simulink model "PolarCinematica"  (R2022a)
settings: Solver=VariableStepAuto  StartTime=0.0  StopTime=Tfinal  RelTol=1e-3
values from neighbouring files (symbols this model uses):
  Tem = 0.001    [circular.m]
undefined symbols (not defined in the file or in its folder): Diferencia, mgd_Polar, mgi_Polar
settings Model: Creator=Shadow  LastModifiedBy=Shadow
settings DebuggingCC: UnconnectedInputMsg=warning  UnconnectedOutputMsg=warning  UnconnectedLineMsg=warning
settings RTWCC: DLArmComputeVersion=19.05

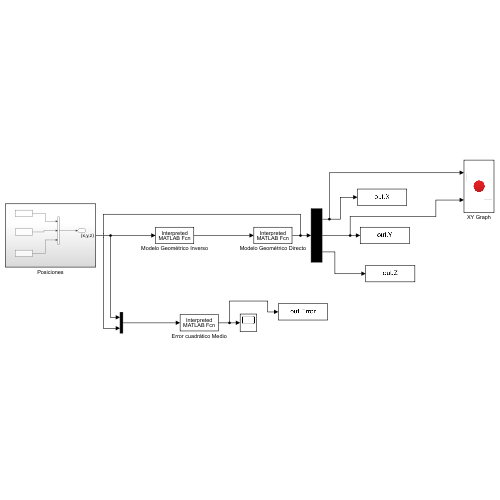
[thumbnail: Simulink's stored preview of the top-level diagram]
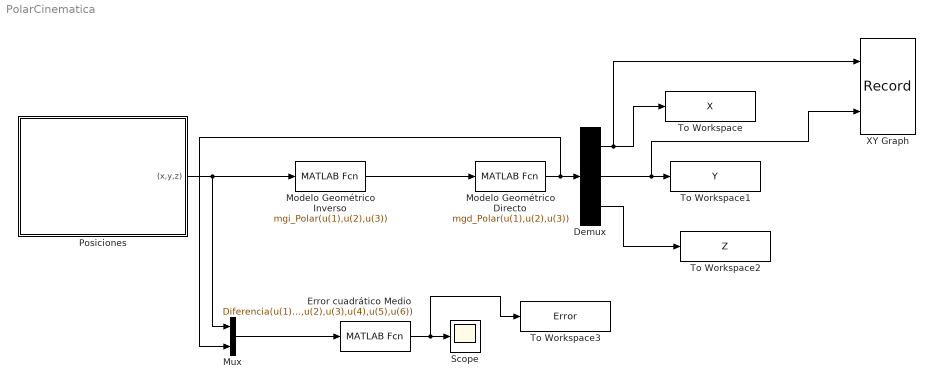
== system PolarCinematica ==
  Demux : Demux  Outputs=3
  Error cuadrático Medio : MATLABFcn  MATLABFcn=Diferencia(u(1),u(2),u(3),u(4),u(5),u(6))  OutputDimensions=1
  Modelo Geométrico Directo : MATLABFcn  MATLABFcn=mgd_Polar(u(1),u(2),u(3))  OutputDimensions=3
  Modelo Geométrico Inverso : MATLABFcn  MATLABFcn=mgi_Polar(u(1),u(2),u(3))  OutputDimensions=3
  Mux : Mux  Inputs=2
  Posiciones : Subsystem
  Scope : Scope
  To Workspace : ToWorkspace  VariableName=X
  To Workspace1 : ToWorkspace  VariableName=Y
  To Workspace2 : ToWorkspace  VariableName=Z
  To Workspace3 : ToWorkspace  VariableName=Error
  XY Graph : Record  FileSettingsInternal="{\"entries\":[{\"content\":{\"excelSettings\":{\"content\":{},\"type\":\"Streamout.ExcelSettings\"}},\"type\":\"Streamout.FileSettingStorage\",\"uuid\":\"bcd1633b-806b-4dc5-b82f-7056fa3f72c6\"}],\"packageUris\":[\"http://schema.mathworks.com/mf0/streamout_blocks/R2020a\"],\"version\":\"1.0\"}"  Layout=[1 1]  SignalsInternal="{\"entries\":[{\"content\":{\"signals\":[{\"content\":{\"blockPath\":[\"PolarCinematica/XY Graph\"],\"channel\":[],\"dimensions\":[1],\"domain\":\"PolarCinematica/XY Graph\",\"lineColor\":\"#a2142f\",\"plots\":[1],\"port\":1,\"sid\":[\"\"],\"signalID\":28,\"signalName\":\"Demux:1\"},\"type\":\"RecordBlkView.Signal\",\"uuid\":\"7db50e9b-d9aa-4afa-8b6e-b476f31eaf6f\"},{\"content\":{\"blockPath\":[\"PolarCinematica/XY Graph\"],\"channel\":[],\"dimensions\":[1],\"domain\":\"PolarCinematica/XY Graph\",\"lineColor\":\"#139fff\",\"plots\":[1],\"port\":2,\"sid\":[\"\"],\"signalID\":32,\"signalName\":\"Demux:2\"},\"type\":\"RecordBlkView.Signal\",\"uuid\":\"48e31d0b-9318-448c-a423-086d85bbcbc5\"}]},\"type\":\"RecordBlkView.InputSignals\",\"uuid\":\"946ceb7c-b64a-43a8-9baa-8683f0c128d2\"}],\"packageUris\":[\"http://schema.mathworks.com/mf0/streamout_blocks/R2020a\"],\"version\":\"1.0\"}"  VisualizationBindings="{\"xyplotplugin\":{\"info\":[{\"series\":[{\"bindingParametersList\":[{\"parameter\":\"X-Axis\",\"signalID\":28,\"signalName\":\"Demux:1\"},{\"parameter\":\"Y-Axis\",\"signalID\":32,\"signalName\":\"Demux:2\"}],\"seriesID\":43994}],\"subplotID\":1}]}}"  CompatibilityTag=XY
  wires:
  Demux/2 -> XY Graph/2, To Workspace1/1
  Demux/3 -> To Workspace2/1
  Modelo Geométrico Inverso/1 -> Modelo Geométrico Directo/1
  Posiciones/1((x,y,z)) -> Mux/1, Modelo Geométrico Inverso/1
  Demux/1 -> To Workspace/1, XY Graph/1
  Mux/1 -> Error cuadrático Medio/1
  Modelo Geométrico Directo/1 -> Mux/2, Demux/1
  Error cuadrático Medio/1 -> To Workspace3/1, Scope/1

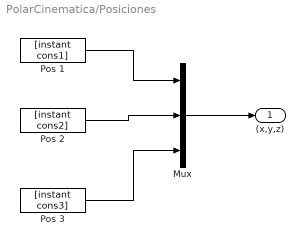
== system PolarCinematica/Posiciones ==
  Mux : Mux  Inputs=3
  Pos 1 : FromWorkspace  VariableName=[instant cons1]  SampleTime=Tem
  Pos 2 : FromWorkspace  VariableName=[instant cons2]  SampleTime=Tem
  Pos 3 : FromWorkspace  VariableName=[instant cons3]  SampleTime=Tem
  (x,y,z) : Outport
  wires:
  Pos 3/1 -> Mux/3
  Pos 1/1 -> Mux/1
  Pos 2/1 -> Mux/2
  Mux/1 -> (x,y,z)/1
